simulink model "thermal_closed_loop_model"  (R2023a)
settings: Solver=VariableStepAuto  StartTime=0.0  StopTime=600  RelTol=1e-3
PostLoadFcn:
  | run('thermal_model_parameters.m')
  | run('thermal_harness_parameters.m')
  | run('thermal_variants_config.m')
values from neighbouring files (symbols this model uses):
  air_cp = 1004    [thermal_harness_parameters.m]
  air_HC_min = 10    [thermal_harness_parameters.m]
  air_HC_nom = 100    [thermal_harness_parameters.m]
  air_rho = 1.2    [thermal_harness_parameters.m]
  air_vel_nom = 1    [thermal_harness_parameters.m]
  coolant_initial_pressure = 0.111325    [thermal_model_parameters.m]    (also in thermal_plant_h2f175_parameters.m)
  coolant_initial_temperature = 293.15    [thermal_model_parameters.m]    (also in thermal_plant_h2f175_parameters.m)
  coolant_tube_D = 0.05    [thermal_model_parameters.m]    (also in thermal_plant_h2f175_parameters.m)
  radiator_area_air = radiator_n_fins * radiator_fin_height * radiator_fin_width    (= 0.1026)    [thermal_harness_parameters.m]
  radiator_area_fins = radiator_n_fins * (radiator_fin_height-radiator_fin_thickness) * radiator_width * 2    (= 2.543625)    [thermal_harness_parameters.m]
  radiator_area_primary = 2 * radiator_tube_length * radiator_width * (radiator_fin_rows)     - 2 * radiator_fin_thickness * radiator_width * radiator_n_fins     + 2 * radiator_fin_height * radiator_width * radiator_fin_rows     + 2 * radiator_tube_height * radiator_n_tubes * radiator_tube_length    [thermal_harness_parameters.m]
  radiator_n_tubes = 20    [thermal_harness_parameters.m]
  radiator_tube_height = 0.0015    [thermal_harness_parameters.m]
  radiator_tube_length = 0.45    [thermal_harness_parameters.m]
  radiator_width = 0.025    [thermal_harness_parameters.m]
  tcp_time_constant = 2    [thermal_model_parameters.m]    (also in thermal_plant_h2f175_parameters.m)
undefined symbols (not defined in the file or in its folder): sigbuilder_block, stack
libraries: fl_lib x35, nesl_utility x23, SimscapeFluids_lib x5, simulink x1
(part 2 of 2)

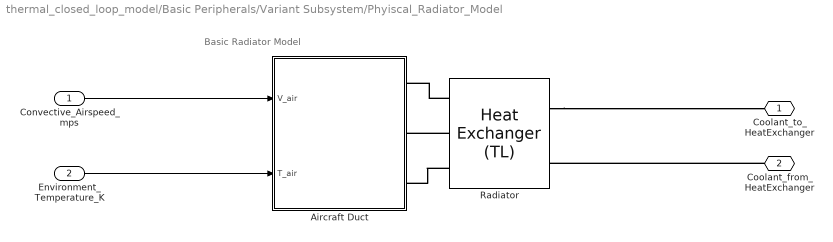
== system thermal_closed_loop_model/Basic Peripherals/Variant Subsystem/Phyiscal_Radiator_Model ==
  note: Basic Radiator Model
  Convective_Airspeed_mps : Inport
  Environment_Temperature_K : Inport  Port=2
  Aircraft Duct : Subsystem
  Radiator : SimscapeFluids_lib/Fluid Network Interfaces/Heat Exchangers/Heat Exchanger (TL)  hex_type=3  shell_num=1  cross_type=4  NTU_TLU=[0.5, 1.0, 2.0, 3.0, 4.0, 5.0]  CR_TLU=[0.0, 0.25, 0.5, 0.75, 1.0]  eff_TLU=[0.3, 0.3, 0.3, 0.3, 0.3; 0.6, 0.55, 0.5, 0.47, 0.43; 0.85, 0.76, 0.68, 0.61, 0.55; 0.94, 0.83, 0.72, 0.65, 0.58; 0.98, 0.86, 0.75, 0.66, 0.58; 0.99, 0.86, 0.75, 0.66, 0.58]  R_wall=0.014/(381*radiator_n_tubes*radiator_width*radiator_tube_length) K/W  min_flow_area_1=radiator_n_tubes*(radiator_width*radiator_tube_height) m^2  Dh_press_1=4*(radiator_width*radiator_tube_height)/(2 * (radiator_width+radiator_tube_height)) m  liquid_volume_1=radiator_n_tubes*(radiator_width*radiator_tube_height)*radiator_tube_length m^3  Re_lam_1=2000  Re_tur_1=4000  pressure_loss_spec_1=fluids.interfaces.enum.pressure_loss_spec.tube_correlation  pressure_loss_coeff_1=15  length_press_1=radiator_tube_length m  length_add_1=0.1 m  roughness_1=15e-6 m  Re_friction_TLU_1=[400.0, 1000.0, 1500.0, 3000.0, 4000.0, 6000.0, 10000.0, 20000.0, 40000.0, 60000.0, 100000.0, 100000000.0]  friction_factor_TLU_1=[0.264, 0.112, 0.071, 0.0417, 0.0387, 0.0268, 0.025, 0.0232, 0.0226, 0.022, 0.0214, 0.0214]  shape_factor_1=64  Re_Euler_TLU_1=[50.0, 500.0, 1000.0, 2000.0]  Euler_TLU_1=[4.4505, 0.6864, 0.4791, 0.3755]  heat_transfer_spec_1=2  heat_transfer_area_1=radiator_n_tubes*2*(radiator_tube_length*radiator_width+radiator_tube_length*radiator_tube_height) m^2  heat_coeff_1=2000 W/(m^2 * K)  length_heat_1=radiator_tube_length cm  Nu_lam_1=3.66  Re_Colburn_TLU_1=[100.0, 150.0, 1000.0]  Colburn_factor_TLU_1=[0.019, 0.013, 0.002]  Re_Nu_TLU_1=[100.0, 150.0, 1000.0]  Pr_Nu_TLU_1=[1.0, 10.0]  Nu_TLU_1=[3.72, 4.21; 3.75, 4.44; 4.21, 7.15]  fouling_factor_1=0 m^2*K/W  min_heat_coeff_1=5 W/(m^2 * K)  heat_transfer_area_2=radiator_area_primary+radiator_area_fins m^2  fouling_factor_2=0 m^2*K/W  min_heat_coeff_2=0.01 W/(m^2 * K)  dynamic_compressibility_1=1  T0_1=coolant_initial_temperature K  p0_1=coolant_initial_pressure MPa  mdot1_TLU=[.1, .2] kg/s  mdot2_TLU=[.2, .3] kg/s  SD_TLU=[35, 35; 50, 50] kW/K  Q_check=1  mdot_dp_TLU_1=[.1, .2] kg/s  p_diff_TLU_1=[.003, .005] MPa  T_ref_in_1=293.15 K  p_ref_in_1=0.101325 MPa  mdot_threshold_1=1e-3 kg/s  area_1=0.01 m^2
      settings: InternalSimscapePortConfiguration="{\"Bottom\":[],\"Left\":[{\"id\":\"A1\",\"label\":\"A1\",\"type\":\"foundation.thermal_liquid.thermal_liquid\"},{\"id\":\"B1\",\"label\":\"B1\",\"type\":\"foundation.thermal_liquid.thermal_liquid\"}],\"Right\":[{\"id\":\"H2\",\"label\":\"H2\",\"type\":\"foundation.thermal.thermal\"},{\"id\":\"C2\",\"label\":\"C2\",\"type\":\"input\"},{\"id\":\"HC2\",\"label\":\"HC2\",\"type\":\"input\"}],\"Top\":[]}"
  Coolant_to_HeatExchanger : PMIOPort  Side=Right
  Coolant_from_HeatExchanger : PMIOPort  Port=2  Side=Right
  wires:
  Environment_Temperature_K/1 -> Aircraft Duct/2(T_air)
  Convective_Airspeed_mps/1 -> Aircraft Duct/1(V_air)
  connections:
  Radiator/RConn1 -- Aircraft Duct/RConn1
  Radiator/RConn2 -- Aircraft Duct/RConn2
  Radiator/LConn1 -- Coolant_to_HeatExchanger/RConn1
  Radiator/RConn3 -- Aircraft Duct/RConn3
  Coolant_from_HeatExchanger/RConn1 -- Radiator/LConn2

== system thermal_closed_loop_model/Basic Peripherals/Variant Subsystem/Controlled_Temperature_HeatExchanger/°C to Kelvin ==
  Temp. (°C) : Inport
  Constant : Constant  Value=273.15
  Sum : Sum  Inputs=|++
  Temp. (K) : Outport
  wires:
  Constant/1 -> Sum/2
  Sum/1 -> Temp. (K)/1
  Temp. (°C)/1 -> Sum/1

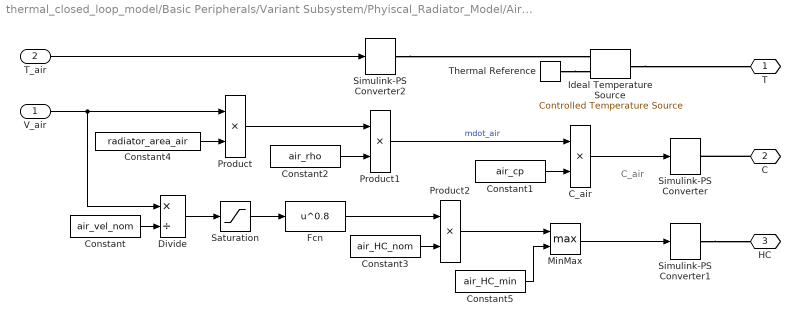
== system thermal_closed_loop_model/Basic Peripherals/Variant Subsystem/Phyiscal_Radiator_Model/Aircraft Duct ==
  note: C_air
  V_air : Inport
  T_air : Inport  Port=2
  C_air : Product
  Constant : Constant  Value=air_vel_nom
  Constant1 : Constant  Value=air_cp
  Constant2 : Constant  Value=air_rho
  Constant3 : Constant  Value=air_HC_nom
  Constant4 : Constant  Value=radiator_area_air
  Constant5 : Constant  Value=air_HC_min
  Divide : Product  Inputs=*/
  Fcn : Fcn  Expr=u^0.8
  Ideal Temperature Source : fl_lib/Thermal/Thermal Sources/Controlled Temperature Source
  MinMax : MinMax  Function=max  Inputs=2
  Product : Product
  Product1 : Product
  Product2 : Product
  Saturation : Saturate  UpperLimit=inf  LowerLimit=0
  Simulink-PS Converter : nesl_utility/Simulink-PS Converter  PhysicalDomain=network_engine_domain  SubClassName=ps_input  LeftPortType=input  RightPortType=output  PseudoPeriodic=off  Frequencies=[]  NoiseDistribution=none  NoiseParameters=[]  Unit=W/K  AffineConversion=off  FilteringAndDerivatives=zero  SimscapeFilterOrder=1  InputFilterTimeConstant=1  UdotUserProvided=1
  Simulink-PS Converter1 : nesl_utility/Simulink-PS Converter  PhysicalDomain=network_engine_domain  SubClassName=ps_input  LeftPortType=input  RightPortType=output  PseudoPeriodic=off  Frequencies=[]  NoiseDistribution=none  NoiseParameters=[]  Unit=W/(m^2*K)  AffineConversion=off  FilteringAndDerivatives=zero  SimscapeFilterOrder=1  InputFilterTimeConstant=1  UdotUserProvided=1
  Simulink-PS Converter2 : nesl_utility/Simulink-PS Converter  PhysicalDomain=network_engine_domain  SubClassName=ps_input  LeftPortType=input  RightPortType=output  PseudoPeriodic=off  Frequencies=[]  NoiseDistribution=none  NoiseParameters=[]  Unit=K  AffineConversion=on  FilteringAndDerivatives=zero  SimscapeFilterOrder=1  InputFilterTimeConstant=1  UdotUserProvided=1
  Thermal Reference : fl_lib/Thermal/Thermal Elements/Thermal Reference
  T : PMIOPort  Side=Right
  C : PMIOPort  Port=2  Side=Right
  HC : PMIOPort  Port=3  Side=Right
  wires:
  V_air/1 -> Product/1, Divide/1
  Constant/1 -> Divide/2
  Constant3/1 -> Product2/2
  Divide/1 -> Saturation/1
  Fcn/1 -> Product2/1
  Product2/1 -> MinMax/1
  Constant5/1 -> MinMax/2
  MinMax/1 -> Simulink-PS Converter1/1
  T_air/1 -> Simulink-PS Converter2/1
  Constant1/1 -> C_air/2
  C_air/1 -> Simulink-PS Converter/1
  Product/1 -> Product1/1
  Constant2/1 -> Product1/2
  Constant4/1 -> Product/2
  Product1/1 -> C_air/1  "mdot_air"
  Saturation/1 -> Fcn/1
  connections:
  C/RConn1 -- Simulink-PS Converter/RConn1
  Simulink-PS Converter1/RConn1 -- HC/RConn1
  Thermal Reference/LConn1 -- Ideal Temperature Source/RConn2
  Simulink-PS Converter2/RConn1 -- Ideal Temperature Source/RConn1
  Ideal Temperature Source/LConn1 -- T/RConn1
